simulink model "Convolution_Ex4"  (R2025a)
settings: Solver=VariableStepAuto  StartTime=0.0  StopTime=512/100e6  RelTol=1e-3
InitFcn:
  | RTP_F = 48;
  | RTP_G = 32;
  | 
  | F_Length = 112;
  | G_Length = 80;
undefined symbols (not defined in the file): Correlation_ValidMode, DUT, Full, S, vsva2197, xcvc1902
libraries: aieDSP x1, aieUtilities x1, vmcUtilities x1
settings Model: Creator=sdegala  LastModifiedBy=sdegala
settings ModelReferenceCC: EnableRefExpFcnMdlSchedulingChecks=on
settings RTWCC: GPUComputeCapability=3.5

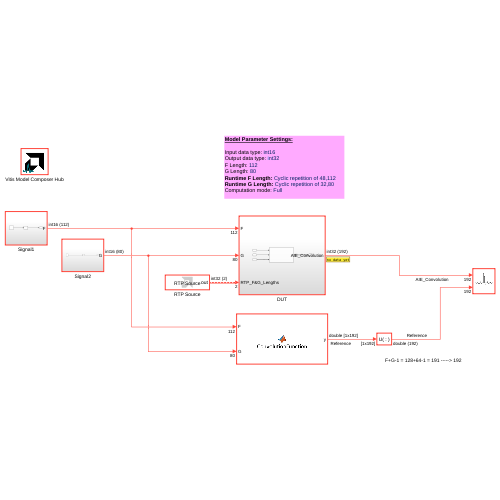
[thumbnail: Simulink's stored preview of the top-level diagram]
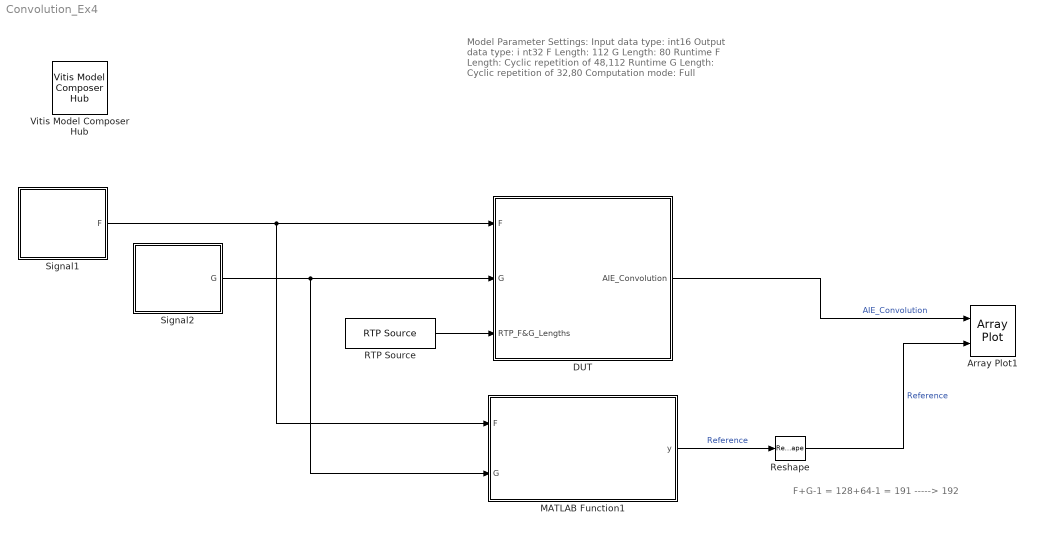
== system Convolution_Ex4 ==
  note: F+G-1 = 128+64-1 = 191 -----> 192
  note: Model Parameter Settings:
      |
      | Input data type: int16
      | Output data type: i nt32
      | F Length: 112
      | G Length: 80
      | Runtime F Length: Cyclic repetition of 48,112
      | Runtime G Length: Cyclic repetition of 32,80
      | Computation mode: Full
  Array Plot1 : ArrayPlot  NumInputPorts=2  WindowPosition=[713.000000,224.000000,1031.000000,765.000000,]  Visible=on  ScopeFrameLocation=window  LayoutDimensions=[1 1]  YLimits=[-2107.375 18966.375]  ShowLegend=on
  DUT : Subsystem
  MATLAB Function1 : MATLAB Function  TreatAsAtomicUnit=on
  RTP Source : aieUtilities/RTP Source  Value=[int32([RTP_F,RTP_G]'),int32([F_Length,G_Length]')]  SampleTime=-1  OutputForm=Cyclic repetition
  Reshape : Reshape
  Signal1 : Subsystem
  Signal2 : Subsystem
  Vitis Model Composer Hub : vmcUtilities/Vitis Model Composer Hub  Tag=genX  CodeGeneration=off  SubsystemName=DUT  BlockHierPath=Correlation_ValidMode/DUT  SubsystemType=AIENode  StartColumn=1  NumberOfColumns=1  TargetDirectory=./code  exportDesign=off  analyzeDesign=on  validateDesignOnHw=off  ExportType=AI Engines  IpVendor=xilinx.com  IpLibrary=hls  IpVersion=1.0  IpHWLanguage=Verilog  AieCompilerOptions={}  AieSimulatorOptions={}  CreateTestbench=on  TestbenchStackSize=10  RunRtlSim=off  RunCSim=off  RunAieSim=off  enableSimulationTimeout=on  enableGraphIterations=on  AieSimTimeout=50000  AieGraphIterations=-1  RunAieSimProfiling=off  LaunchVitisAnalyzer=off  PlotOutput=off  RunX86Sim=off  X86SimTimeout=10  GenHwImage=off  GenLibadfXo=off  GenHwValidationCode=off  PlatformType=Not Specified  HwSystemType=Baremetal  HwValidationTarget=hw  ProjDevice=xcvc1902-vsva2197-1LP-e-S  ProjDevicePart=xcvc1902-vsva2197-1LP-e-S  AIEType=AIE  SamplePeriod=-1  ClockFrequency=200  DataPathParallelism=1  xilinxfamily=versalaicore  part=xcvc1902  speed=-1LP-e-S  package=vsva2197  directory=./netlist  testbench=off  incr_netlist=off  synthesis_tool=Vivado  clock_wrapper=Clock Enables  dbl_ovrd=According to Block Masks  dcm_input_clock_period=10  sysclk_period=10  simulink_period=1  eval_field=0  IPInfoJsonString="{\"DUTSubsystemName\":\"DUT\",\"AIESubsystem\":{\"SubsystemName\":\"DUT\",\"TargetDirectory\":\"./code\",\"AIEArrayConfig\":\"Use entire AIE array\",\"StartColumn\":\"0\",\"NumberOfColumns\":\"1\"},\"SubsystemTag\":\"AIENode\"}"  LogFileName=/proj/xhdhdstaff5/sdegala/Head1/HEAD/2025_2_work/AIE_BLOCKS_2025_2/code/model_composer.log  NThreads=4  IPConfigFile=/tmp/vmctmp-11198269997411262707/Correlation_ValidMode_ipconfig.json
  wires:
  RTP Source/1 -> DUT/3(RTP_F&G_Lengths)
  Signal2/1(G) -> DUT/2(G), MATLAB Function1/2(G)
  Signal1/1(F) -> DUT/1(F), MATLAB Function1/1(F)
  MATLAB Function1/1(y) -> Reshape/1  "Reference"
  Reshape/1 -> Array Plot1/2  "Reference"
  DUT/1(AIE_Convolution) -> Array Plot1/1  "AIE_Convolution"

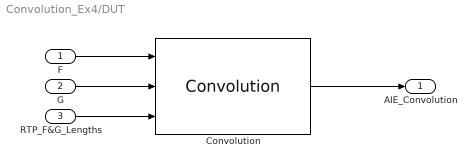
== system Convolution_Ex4/DUT ==
  F : Inport
  G : Inport  Port=2
  RTP_F&G_Lengths : Inport  Port=3
  Convolution : aieDSP/Convolution  AIE_VARIANT=1  api=0  data_type_f=int16  data_type_g=int16  data_type_out=int32  function_type=1  compute_mode=Full (0)  f_sample_size=F_Length  g_sample_size=G_Length  USE_RTP_VECTOR_LENGTHS=on  num_frames=1  shift_output=0  rnd_mode=Floor  sat_mode=None  no_of_kernels=1  casc_length=1  blockJsonConstraints=[]  blockJsonConstraintsInternal=[]  spec=vmc_conv.json  SerializedMaskParamNames=[]  SerializedMaskParamValues=[]  SerializedMaskParamVisibilities=[]  block_type=Convolution  SerializedMaskParamDataypes=uint|uint|typename|typename|typename|uint|uint|uint|uint|uint|uint|uint|uint|uint|uint|uint  SerializedMaskParamEnumStrArr=0|0|0|0|0|0|Full (0),Same (1),Valid (2)|0|0|0|0|0|Floor,Ceiling,Round to positive infinity,Round to negative infinity,Round symmetrical to infinity,Round symmetrical to zero,Round convergent to even,Round convergent to odd|None,Saturate,Symmetric|0|0  SerializedMaskParamEnumValArr=0|0|0|0|0|0|0,1,2|0|0|0|0|0|0,1,2,3,4,5,6,7|0,1,3|0|0  SerializedMaskParamVectorArr=0|0|0|0|0|0|0|0|0|0|0|0|0|0|0|0  SerializedMaskParamKeys=AIE_VARIANT|TP_API|TT_DATA_F|TT_DATA_G|TT_DATA_OUT|TP_FUNCT_TYPE|TP_COMPUTE_MODE|TP_F_LEN|TP_G_LEN|TP_USE_RTP_VECTOR_LENGTHS|TP_NUM_FRAMES|TP_SHIFT|TP_RND|TP_SAT|TP_PHASES|TP_CASC_LEN
  AIE_Convolution : Outport
  wires:
  F/1 -> Convolution/1
  G/1 -> Convolution/2
  Convolution/1 -> AIE_Convolution/1
  RTP_F&G_Lengths/1 -> Convolution/3

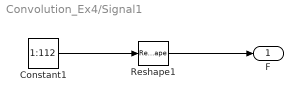
== system Convolution_Ex4/Signal1 ==
  Constant1 : Constant  Value=1:112  OutDataTypeStr=int16  SampleTime=1/100e6
  Reshape1 : Reshape
  F : Outport
  wires:
  Reshape1/1 -> F/1
  Constant1/1 -> Reshape1/1

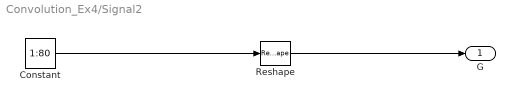
== system Convolution_Ex4/Signal2 ==
  Constant : Constant  Value=1:80  OutDataTypeStr=int16  SampleTime=1/100e6
  Reshape : Reshape
  G : Outport
  wires:
  Reshape/1 -> G/1
  Constant/1 -> Reshape/1

== matlab function Convolution_Ex4/MATLAB Function1 ==
  data: F input; G input; y output
function y = ConvolutionFunction(F, G)


persistent i
if isempty(i), i = uint32(0); end

i = i + 1;


 % % Normalize to row vectors
 %    F = F(:).'; 
 %    G = G(:).';
y = zeros(1,112+80); % F_Length+G_Length = 128+64

if mod(i,2) == 0

        RTP_F_Length = 112;
        RTP_G_Length = 80;
else

        RTP_F_Length = 48;
        RTP_G_Length = 32;
end

y(1:RTP_F_Length+RTP_G_Length-1) = conv(F(1:RTP_F_Length),G(1:RTP_G_Length),'full'); 


end
